simulink model "StateflowKalman"  (R2017a)
settings: Solver=FixedStepDiscrete  StartTime=0.0  StopTime=inf  FixedStep=0.001  RelTol=1e-3  EnableMultiTasking=on
values from neighbouring files (symbols this model uses):
  C = B    [testMatricePiccola.m]
undefined symbols (not defined in the file or in its folder): DiscIntNeverNeededParam, Discrete, Time
libraries: xpcethercatlib x29, simulink x14, powerlib_meascontrol x3, commutil2 x2, ctrlSharedLib x2, simulink_extras x2
(part 3 of 3)

== matlab function StateflowKalman/Sistema_braccia/Cinematica Inversa Acc ==
  data: x input; y input; x_p input; y_p input; x_pp input; y_pp input; theta1 input; theta2 input; theta1_pp output; theta1_p input; theta2_p input; theta2_pp output
function [theta1_pp, theta2_pp] = CinInvAcc(x, y, x_p, y_p, x_pp, y_pp, theta1, theta2, theta1_p,theta2_p)

d = 0.09; 
l = 0.25;

N21 = -l*sin(theta1)*(x+d-l*cos(theta1)) + l*cos(theta1)*(y-l*sin(theta1));

N22 = -l*cos(theta2)*(y-l*sin(theta2))*(x+d-l*cos(theta1))/(x-d-l*cos(theta2)) + l*sin(theta2)*(x+d-l*cos(theta1));

D2 = y-l*sin(theta1) - (y-l*sin(theta2))*(x+d-l*cos(theta1))/(x-d-l*cos(theta2));

J21 = N21/D2;

J22 = N22/D2;

J11 = -(y-l*sin(theta2))/(x-d-l*cos(theta2))*(J21);

J12 = -(y-l*sin(theta2))/(x-d-l*cos(theta2))*(J22) -l*sin(theta2) + (y-l*sin(theta2))/(x-d-l*cos(theta2))*(l*cos(theta2));

J = [J11 J12; J21 J22];

J_p11 = ((l*cos(theta1)*(y - l*sin(theta1)) - l*sin(theta1)*(d + x - l*cos(theta1)))*(y_p - l*cos(theta2)*theta2_p))/((d - x + l*cos(theta2))*(y - l*sin(theta1) + ((y - l*sin(theta2))*(d + x - l*cos(theta1)))/(d - x + l*cos(theta2)))) - ((y - l*sin(theta2))*(l*sin(theta1)*(x_p + l*sin(theta1)*theta1_p) - l*cos(theta1)*(y_p - l*cos(theta1)*theta1_p) + l*sin(theta1)*(y - l*sin(theta1))*theta1_p + l*cos(theta1)*theta1_p*(d + x - l*cos(theta1))))/((d - x + l*cos(theta2))*(y - l*sin(theta1) + ((y - l*sin(theta2))*(d + x - l*cos(theta1)))/(d - x + l*cos(theta2)))) + ((x_p + l*sin(theta2)*theta2_p)*(y - l*sin(theta2))*(l*cos(theta1)*(y - l*sin(theta1)) - l*sin(theta1)*(d + x - l*cos(theta1))))/((d - x + l*cos(theta2))^2*(y - l*sin(theta1) + ((y - l*sin(theta2))*(d + x - l*cos(theta1)))/(d - x + l*cos(theta2)))) - ((y - l*sin(theta2))*(l*cos(theta1)*(y - l*sin(theta1)) - l*sin(theta1)*(d + x - l*cos(theta1)))*(y_p + ((x_p + l*sin(theta1)*theta1_p)*(y - l*sin(theta2)))/(d - x + l*cos(theta2)) + ((y_p - l*cos(theta2)*theta2_p)*(d + x - l*cos(theta1)))/(d - x + l*cos(theta2)) - l*cos(theta1)*theta1_p + ((x_p + l*sin(theta2)*theta2_p)*(y - l*sin(theta2))*(d + x - l*cos(theta1)))/(d - x + l*cos(theta2))^2))/((d - x + l*cos(theta2))*(y - l*sin(theta1) + ((y - l*sin(theta2))*(d + x - l*cos(theta1)))/(d - x + l*cos(theta2)))^2);
 
 
J_p12 = ((y - l*sin(theta2))*(l*sin(theta2)*(x_p + l*sin(theta1)*theta1_p) + l*cos(theta2)*theta2_p*(d + x - l*cos(theta1)) + (l*cos(theta2)*(x_p + l*sin(theta1)*theta1_p)*(y - l*sin(theta2)))/(d - x + l*cos(theta2)) + (l*cos(theta2)*(y_p - l*cos(theta2)*theta2_p)*(d + x - l*cos(theta1)))/(d - x + l*cos(theta2)) - (l*sin(theta2)*(y - l*sin(theta2))*theta2_p*(d + x - l*cos(theta1)))/(d - x + l*cos(theta2)) + (l*cos(theta2)*(x_p + l*sin(theta2)*theta2_p)*(y - l*sin(theta2))*(d + x - l*cos(theta1)))/(d - x + l*cos(theta2))^2))/((d - x + l*cos(theta2))*(y - l*sin(theta1) + ((y - l*sin(theta2))*(d + x - l*cos(theta1)))/(d - x + l*cos(theta2)))) - l*cos(theta2)*theta2_p - (l*cos(theta2)*(y_p - l*cos(theta2)*theta2_p))/(d - x + l*cos(theta2)) + ((l*sin(theta2)*(d + x - l*cos(theta1)) + (l*cos(theta2)*(y - l*sin(theta2))*(d + x - l*cos(theta1)))/(d - x + l*cos(theta2)))*(y_p - l*cos(theta2)*theta2_p))/((d - x + l*cos(theta2))*(y - l*sin(theta1) + ((y - l*sin(theta2))*(d + x - l*cos(theta1)))/(d - x + l*cos(theta2)))) - (l*cos(theta2)*(x_p + l*sin(theta2)*theta2_p)*(y - l*sin(theta2)))/(d - x + l*cos(theta2))^2 + ((x_p + l*sin(theta2)*theta2_p)*(l*sin(theta2)*(d + x - l*cos(theta1)) + (l*cos(theta2)*(y - l*sin(theta2))*(d + x - l*cos(theta1)))/(d - x + l*cos(theta2)))*(y - l*sin(theta2)))/((d - x + l*cos(theta2))^2*(y - l*sin(theta1) + ((y - l*sin(theta2))*(d + x - l*cos(theta1)))/(d - x + l*cos(theta2)))) - ((l*sin(theta2)*(d + x - l*cos(theta1)) + (l*cos(theta2)*(y - l*sin(theta2))*(d + x - l*cos(theta1)))/(d - x + l*cos(theta2)))*(y - l*sin(theta2))*(y_p + ((x_p + l*sin(theta1)*theta1_p)*(y - l*sin(theta2)))/(d - x + l*cos(theta2)) + ((y_p - l*cos(theta2)*theta2_p)*(d + x - l*cos(theta1)))/(d - x + l*cos(theta2)) - l*cos(theta1)*theta1_p + ((x_p + l*sin(theta2)*theta2_p)*(y - l*sin(theta2))*(d + x - l*cos(theta1)))/(d - x + l*cos(theta2))^2))/((d - x + l*cos(theta2))*(y - l*sin(theta1) + ((y - l*sin(theta2))*(d + x - l*cos(theta1)))/(d - x + l*cos(theta2)))^2) + (l*sin(theta2)*(y - l*sin(theta2))*theta2_p)/(d - x + l*cos(theta2));
 
 
J_p21 = - (l*sin(theta1)*(x_p + l*sin(theta1)*theta1_p) - l*cos(theta1)*(y_p - l*cos(theta1)*theta1_p) + l*sin(theta1)*(y - l*sin(theta1))*theta1_p + l*cos(theta1)*theta1_p*(d + x - l*cos(theta1)))/(y - l*sin(theta1) + ((y - l*sin(theta2))*(d + x - l*cos(theta1)))/(d - x + l*cos(theta2))) - ((l*cos(theta1)*(y - l*sin(theta1)) - l*sin(theta1)*(d + x - l*cos(theta1)))*(y_p + ((x_p + l*sin(theta1)*theta1_p)*(y - l*sin(theta2)))/(d - x + l*cos(theta2)) + ((y_p - l*cos(theta2)*theta2_p)*(d + x - l*cos(theta1)))/(d - x + l*cos(theta2)) - l*cos(theta1)*theta1_p + ((x_p + l*sin(theta2)*theta2_p)*(y - l*sin(theta2))*(d + x - l*cos(theta1)))/(d - x + l*cos(theta2))^2))/(y - l*sin(theta1) + ((y - l*sin(theta2))*(d + x - l*cos(theta1)))/(d - x + l*cos(theta2)))^2;
 
 
J_p22 = (l*sin(theta2)*(x_p + l*sin(theta1)*theta1_p) + l*cos(theta2)*theta2_p*(d + x - l*cos(theta1)) + (l*cos(theta2)*(x_p + l*sin(theta1)*theta1_p)*(y - l*sin(theta2)))/(d - x + l*cos(theta2)) + (l*cos(theta2)*(y_p - l*cos(theta2)*theta2_p)*(d + x - l*cos(theta1)))/(d - x + l*cos(theta2)) - (l*sin(theta2)*(y - l*sin(theta2))*theta2_p*(d + x - l*cos(theta1)))/(d - x + l*cos(theta2)) + (l*cos(theta2)*(x_p + l*sin(theta2)*theta2_p)*(y - l*sin(theta2))*(d + x - l*cos(theta1)))/(d - x + l*cos(theta2))^2)/(y - l*sin(theta1) + ((y - l*sin(theta2))*(d + x - l*cos(theta1)))/(d - x + l*cos(theta2))) - ((l*sin(theta2)*(d + x - l*cos(theta1)) + (l*cos(theta2)*(y - l*sin(theta2))*(d + x - l*cos(theta1)))/(d - x + l*cos(theta2)))*(y_p + ((x_p + l*sin(theta1)*theta1_p)*(y - l*sin(theta2)))/(d - x + l*cos(theta2)) + ((y_p - l*cos(theta2)*theta2_p)*(d + x - l*cos(theta1)))/(d - x + l*cos(theta2)) - l*cos(theta1)*theta1_p + ((x_p + l*sin(theta2)*theta2_p)*(y - l*sin(theta2))*(d + x - l*cos(theta1)))/(d - x + l*cos(theta2))^2))/(y - l*sin(theta1) + ((y - l*sin(theta2))*(d + x - l*cos(theta1)))/(d - x + l*cos(theta2)))^2;
 

J_p = [J_p11, J_p12
    J_p21, J_p22];
     
Theta_pp = (inv(J))*([x_pp; y_pp] - J_p*[theta1_p; theta2_p]);

theta1_pp = Theta_pp(1,1);
theta2_pp = Theta_pp(2,1);

== matlab function StateflowKalman/Sistema_braccia/Cinematica diretta Acc ==
  data: theta1 input; x_pp output; theta2 input; theta1_p input; theta2_p input; theta1_pp input; theta2_pp input; x input; y input; x_p input; y_p input; y_pp output
function [x_pp, y_pp] = fcn(theta1, theta2, theta1_p, theta2_p, theta1_pp, theta2_pp, x, y, x_p, y_p)

d = 0.09; 
l = 0.25;

A = x_p^2 + 2*l*sin(theta2)*x_p*theta2_p + (l*sin(theta2)*theta2_p)^2 + (x-d-l*cos(theta2))*(l*cos(theta2)*theta2_p^2 + l*sin(theta2)*theta2_pp) +...
    y_p^2 - 2*l*cos(theta2)*y_p*theta2_p + (l*cos(theta2)*theta2_p)^2 + (y-l*sin(theta2))*(l*sin(theta2)*theta2_p^2 - l*cos(theta2)*theta2_pp);

B = x_p^2 + 2*l*sin(theta1)*x_p*theta1_p + (l*sin(theta1)*theta1_p)^2 + (x+d-l*cos(theta1))*(l*cos(theta1)*theta1_p^2 + l*sin(theta1)*theta1_pp) +...
    y_p^2 - 2*l*cos(theta1)*y_p*theta1_p + (l*cos(theta1)*theta1_p)^2 + (y-l*sin(theta1))*(l*sin(theta1)*theta1_p^2 - l*cos(theta1)*theta1_pp);

y_pp = (B*(x-d-l*cos(theta2))/(x+d-l*cos(theta1)) - A)/(y-l*sin(theta2) - (x-d-l*cos(theta2))/(x+d-l*cos(theta1))*(y-l*sin(theta1)));

x_pp = (-y_pp*(y-l*sin(theta1)) - B)/(x+d-l*cos(theta1));

== matlab function StateflowKalman/Sistema_braccia/Velocita /Vel Asse B conv ==
  data: p input; vel_B_conv output
function vel_B_conv = fcn(p)
vel_B_conv = p  *(2*pi)/163840/64;

== matlab function StateflowKalman/Sistema_braccia/Dinamica Inversa1 ==
  data: bool input; theta1 input; C1 output; C2 output; theta2 input; theta1_p input; theta2_p input; theta1_pp input; theta2_pp input; M output; K output
function [C1, C2, M, K] = Dinamica_Inversa(bool, theta1,theta2,theta1_p,theta2_p,theta1_pp,theta2_pp)
d = 0.09;
l = 0.25;
m = 2.9;
me = 0.36;
pv = 0.02;
Jv = 6.4e-06;
J = 5.22e-02;

A1 = cos(theta1)*theta1_p^2 + sin(theta1)*theta1_pp;
A2 = cos(theta2)*theta2_p^2 + sin(theta2)*theta2_pp;
B1 = -sin(theta1)*theta1_p^2 + cos(theta1)*theta1_pp;
B2 = -sin(theta2)*theta2_p^2 + cos(theta2)*theta2_pp;

theta3 = 2*atan((sin(theta2) - sin(theta1) + ((cos(theta2) - cos(theta1) + 18/25)^2 - ((cos(theta2) - cos(theta1) + 18/25)^2/2 +...
    (sin(theta1) - sin(theta2))^2/2)^2 + (sin(theta1) - sin(theta2))^2)^(1/2))/(cos(theta2) - cos(theta1) +...
    (cos(theta2) - cos(theta1) + 18/25)^2/2 + (sin(theta1) - sin(theta2))^2/2 + 18/25));

theta4 = -2*atan((sin(theta2) - sin(theta1) + ((cos(theta2) - cos(theta1) + 18/25)^2 - ((cos(theta2) - cos(theta1) + 18/25)^2/2 + (sin(theta1) -...
    sin(theta2))^2/2)^2 + (sin(theta1) - sin(theta2))^2)^(1/2))/(cos(theta1) - cos(theta2) + (cos(theta2) - cos(theta1) + 18/25)^2/2 +...
    (sin(theta1) -sin(theta2))^2/2 - 18/25));

N13 = cos(theta4)/sin(theta4)*sin(theta1)-cos(theta1);
N23 = cos(theta2)-cos(theta4)/sin(theta4)*sin(theta2);
D13 = cos(theta3)-cos(theta4)/sin(theta4)*sin(theta3);

theta3_p = (theta1_p*(N13)+theta2_p*(N23))/D13;

N21 = sin(theta1)*(cos(theta3)/sin(theta3) - cos(theta4)/sin(theta4)) +...
    cos(theta4)/sin(theta4)*sin(theta1) - cos(theta1);
N22 = -sin(theta2)*(cos(theta3)/sin(theta3) - cos(theta4)/sin(theta4)) -...
    cos(theta4)/sin(theta4)*sin(theta2) + cos(theta2);
D2 = sin(theta4)*(cos(theta3)/sin(theta3) - cos(theta4)/sin(theta4));

theta4_p = theta1_p*(N21/D2)+ theta2_p*(N22/D2);

J34 = [N13/D13, N23/D13; N21/D2, N22/D2];

theta3_pp = (-B1 +B2 + sin(theta3)*theta3_p^2 - sin(theta4)*theta4_p^2 + cos(theta4)/sin(theta4)*(A1 - A2 + cos(theta3)*theta3_p^2 - cos(theta4)*theta4_p^2))/...
    (cos(theta3) - cos(theta4)/sin(theta4)*sin(theta3));

theta4_pp = (A1 - A2 + cos(theta3)*theta3_p^2 - cos(theta4)*theta4_p^2 + sin(theta3)*theta3_pp)/sin(theta4);

N11 = cos(theta4)/sin(theta4)*sin(theta1)-cos(theta1);
N12 = cos(theta2)-cos(theta4)/sin(theta4)*sin(theta2);
D1 = cos(theta3)-cos(theta4)/sin(theta4)*sin(theta3);

N21 = sin(theta1)*(cos(theta3)/sin(theta3) - cos(theta4)/sin(theta4)) +...
    cos(theta4)/sin(theta4)*sin(theta1) - cos(theta1);
N22 = -sin(theta2)*(cos(theta3)/sin(theta3) - cos(theta4)/sin(theta4)) -...
    cos(theta4)/sin(theta4)*sin(theta2) + cos(theta2);
D2 = sin(theta4)*(cos(theta3)/sin(theta3) - cos(theta4)/sin(theta4));

N11p =  (-1)/(sin(theta4)^2)*theta4_p*sin(theta1) + cos(theta4)/sin(theta4)*cos(theta1)*theta1_p + sin(theta1)*theta1_p;

N12p = -(-1)/(sin(theta4)^2)*theta4_p*sin(theta2) - cos(theta4)/sin(theta4)*cos(theta2)*theta2_p - sin(theta2)*theta2_p;

D1p = -sin(theta3)*theta3_p -(-1)/(sin(theta4)^2)*theta4_p*sin(theta3) - cos(theta4)/sin(theta4)*cos(theta3)*theta3_p;

N21p = cos(theta1)*theta1_p*(cos(theta3)/sin(theta3) - cos(theta4)/sin(theta4)) + sin(theta1)*((-1)/(sin(theta3)^2)*theta3_p + 1/(sin(theta4)^2)*theta4_p) + ...
    (-1)/(sin(theta4)^2)*theta4_p*sin(theta1) + cos(theta4)/sin(theta4)*cos(theta1)*theta1_p + sin(theta1)*theta1_p;

N22p = -cos(theta2)*theta2_p*(cos(theta3)/sin(theta3) - cos(theta4)/sin(theta4)) - sin(theta2)*((-1)/(sin(theta3)^2)*theta3_p + 1/(sin(theta4)^2)*theta4_p) - ...
    (-1)/(sin(theta4)^2)*theta4_p*sin(theta2) - cos(theta4)/sin(theta4)*cos(theta2)*theta2_p - sin(theta2)*theta2_p;

D2p = cos(theta4)*theta4_p*(cos(theta3)/sin(theta3) - cos(theta4)/sin(theta4)) + sin(theta4)*((-1)/(sin(theta3)^2)*theta3_p + 1/(sin(theta4)^2)*theta4_p);

J34p = [(N11p*D1 - N11*D1p)/(D1^2), (N12p*D1 - N12*D1p)/(D1^2);(N21p*D2 - N21*D2p)/(D2^2), (N22p*D2 - N22*D2p)/(D2^2)];

J1 = [-0.5*l*sin(theta1), 0;
        0.5*l*cos(theta1), 0]; 
J1p = [-0.5*l*cos(theta1)*theta1_p, 0;
       -0.5*l*sin(theta1)*theta1_p, 0];

J2 = [0, -0.5*l*sin(theta2);
       0,  0.5*l*cos(theta2)]; 
J2p = [0, -0.5*l*cos(theta2)*theta2_p;
       0, -0.5*l*sin(theta2)*theta2_p];

J3 = [ -l*(sin(theta1)+0.5*sin(theta3)*J34(1,1)), -l*(0.5*sin(theta3)*J34(1,2));
        l*(cos(theta1)+0.5*cos(theta3)*J34(1,1)),  l*(0.5*cos(theta3)*J34(1,2))];
J3p = [ -l*(cos(theta1)*theta1_p+0.5*cos(theta3)*theta3_p*J34(1,1)+0.5*sin(theta3)*J34p(1,1)), -l*(0.5*cos(theta3)*theta3_p*J34(1,2)+0.5*sin(theta3)*J34p(1,2));
        l*(-sin(theta1)*theta1_p-0.5*sin(theta3)*theta3_p*J34(1,1)+0.5*cos(theta3)*J34p(1,1)), l*(-0.5*sin(theta3)*theta3_p*J34(1,2)+0.5*cos(theta3)*J34p(1,2))];

J4 = [ -l*0.5*sin(theta4)*J34(2,1), -l*(sin(theta2)+0.5*sin(theta4)*J34(2,2));
         l*0.5*cos(theta4)*J34(2,1),  l*(cos(theta2)+0.5*cos(theta4)*J34(2,2))];
J4p = [ -l*(0.5*cos(theta4)*theta4_p*J34(2,1)+0.5*sin(theta4)*J34p(2,1)), -l*(cos(theta2)*theta2_p+0.5*cos(theta4)*theta4_p*J34(2,2)+0.5*sin(theta4)*J34p(2,2));
        l*(-0.5*sin(theta4)*theta4_p*J34(2,1)+0.5*cos(theta4)*J34p(2,1)), l*(-sin(theta2)*theta2_p-0.5*sin(theta4)*theta4_p*J34(2,2)+0.5*cos(theta4)*J34p(2,2))];

JE = [ -l*(sin(theta1)+sin(theta3)*J34(1,1)), -l*(sin(theta3)*J34(1,2));
        l*(cos(theta1)+cos(theta3)*J34(1,1)),  l*(cos(theta3)*J34(1,2))];
JEp = [ -l*(cos(theta1)*theta1_p+cos(theta3)*theta3_p*J34(1,1)+sin(theta3)*J34p(1,1)), -l*(cos(theta3)*theta3_p*J34(1,2)+sin(theta3)*J34p(1,2));
        l*(-sin(theta1)*theta1_p-sin(theta3)*theta3_p*J34(1,1)+cos(theta3)*J34p(1,1)), l*(-sin(theta3)*theta3_p*J34(1,2)+cos(theta3)*J34p(1,2))];
  
  
M = (J*eye(2) + m*(J1')*J1 + m*(J2')*J2 + J*(J34')*J34 + m*(J3')*J3 + m*(J4')*J4 + me*(JE')*JE);
K = (m*(J1')*J1p + m*(J2')*J2p + J*(J34')*J34p + m*(J3')*J3p + m*(J4')*J4p + me*(JE')*JEp);

C = M*[theta1_pp; theta2_pp] + K*[theta1_p; theta2_p];

Jm = [1.7e-05, 0; 0, 1.7e-05];
Jtrasm = [1/64, 0; 0, 1/64];
Thetam_pp = Jtrasm^-1*[theta1_pp; theta2_pp];
Thetam_p = Jtrasm^-1*[theta1_p; theta2_p];


% Cm = Jtrasm*C + Jm*Thetam_pp;
Mm = (Jtrasm'*M*Jtrasm + Jm);

    
Km = (Jtrasm'*K*Jtrasm);
nhat = 1e-03*[0.2485; -0.2483];
nm =  Km*Thetam_p;
ntilde = norm(nhat-nm);

% 
% Mm_ = Jm;
% DMm = Mm-Jm;
% D = DMm*Thetam_pp + Km*Thetam_p;
% Aol = [zeros(2,2) eye(2,2); zeros(2,2), zeros(2,2)];
% Bt = [zeros(2,2); Mm_^-1];
% Acl = Aol - Bt*[Kp Kd];


C1 = C(1,1);
C2 = C(2,1);

== matlab function StateflowKalman/Sistema_braccia/Velocita braccia 1/Vel Asse A conv ==
  data: vA input; vel_A_conv output
function vel_A_conv = fcn(vA)
vel_A_conv = (vA)  *(2*pi)/163840/64;

== matlab function StateflowKalman/Sistema_braccia/Posizioni/Asse B conv brac1 ==
  data: p input; pos_B_conv output
function pos_B_conv = fcn(p)
pos_B_conv = p * (2*pi)/16384/64;

== matlab function StateflowKalman/Sistema_braccia/Posizioni/Asse A conv bracc ==
  data: p input; pos_A_conv output
function pos_A_conv = fcn(p)
pos_A_conv = p * (2*pi)/16384/64;

== matlab function StateflowKalman/Sistema_braccia/Velocita braccia 1/Vel Asse B conv ==
  data: p input; vel_B_conv output
function vel_B_conv = fcn(p)
vel_B_conv = p  *(2*pi)/163840/64;

== matlab function StateflowKalman/Sistema_braccia/MATLAB Function2 ==
  data: x input; xp output; y input; yp output; bool input
function [xp,yp] = fcn(x, y, bool)
if bool == 4
    xp = x;
    yp = y;
else
    xp = 0;
    yp = 0;
end

== matlab function StateflowKalman/Sistema_braccia/Coppia motrice ==
  data: Cr1 input; Cm1 output; Cr2 input; theta1_pp input; theta2_pp input; Cm2 output
function [Cm1, Cm2] = fcn(Cr1, Cr2, theta1_pp, theta2_pp)
Jm = 1.7e-05;
i = 64;
Cm1 = (Cr1 + Jm*i^2*theta1_pp)/i;
Cm2 = (Cr2 + Jm*i^2*theta2_pp)/i;
